simulink model "Temp"  (R2018a)
settings: Solver=FixedStepAuto  StartTime=0.0  StopTime=100  FixedStep=10^-2  RelTol=1e-3
values from neighbouring files (symbols this model uses):
  Af = 80 - ABS_ZERO_TEMP    (= 353.15)    [TempBris.m]    (also in TensileSMA.m = 353)
  As = 70 - ABS_ZERO_TEMP    (= 343.15)    [TempBris.m]    (also in TensileSMA.m = 343)
  austeniteLatentCoef = 12188    [TempBris.m]
  BOLTZ_CONST = 5.6703 * 10^-8    (= 5.6703e-08)    [TempBris.m]
  emissivity = 0.75    [TempBris.m]
  Mf = 40 - ABS_ZERO_TEMP    (= 313.15)    [TempBris.m]    (also in TensileSMA.m = 313)
  Ms = 50 - ABS_ZERO_TEMP    (= 323.15)    [TempBris.m]    (also in TensileSMA.m = 323)
  resistanceAustenite = 4 * pi * wireLength * austeniteResistivity / wireDiameter^2    (= 11.5409547722)    [TempBris.m]
  resistanceMartensite = 4 * pi * wireLength * martensiteResistivity / wireDiameter^2    (= 10.6964946669)    [TempBris.m]
  specificHeat = 465.2    [TempBris.m]
  tempEnd = 80 + 273    (= 353)    [TempBris.m]
  tempStart = 80 + 273    (= 353)    [TempBris.m]
  voltage = 2    [TempBris.m]
  wireMass = wireVolume * density    (= 2.21629544234e-05)    [TempBris.m]
  wireSurfaceArea = wireLength * pi * wireDiameter    (= 5.49778714378e-05)    [TempBris.m]
libraries: simulink x3
settings Model: Creator=Michau  LastModifiedBy=Michau

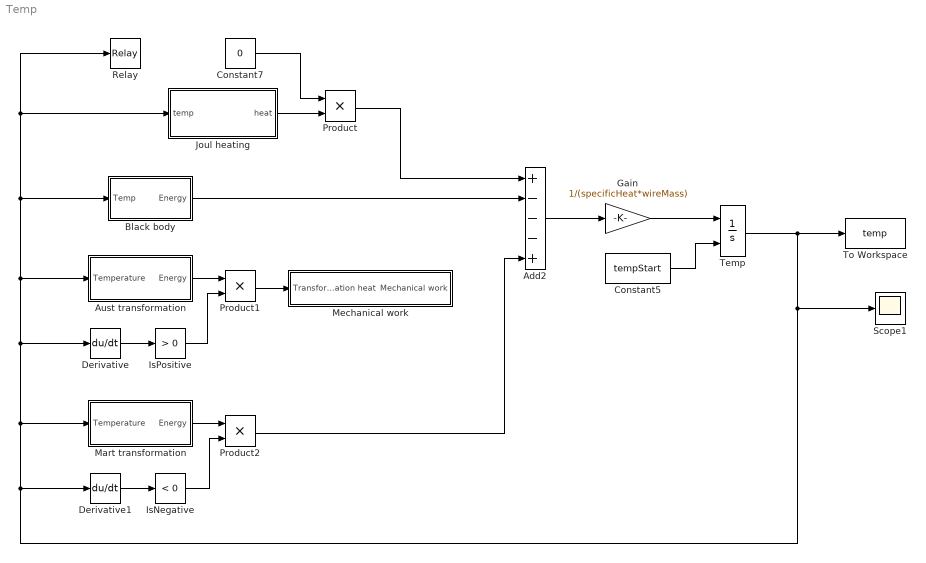
== system Temp ==
  Add2 : Sum  Inputs=+---+
  Aust transformation : Subsystem
  Black body : Subsystem
  Constant5 : Constant  Value=tempStart
  Constant7 : Constant  Value=0
  Derivative : Derivative
  Derivative1 : Derivative
  Gain : Gain  Gain=1/(specificHeat*wireMass)
  IsNegative : simulink/Logic and Bit Operations/Compare To Zero  relop=<  OutDataTypeStr=boolean
  IsPositive : simulink/Logic and Bit Operations/Compare To Zero  relop=>  OutDataTypeStr=boolean
  Joul heating : Subsystem
  Mart transformation : Subsystem
  Mechanical work : Subsystem
  Product : Product
  Product1 : Product
  Product2 : Product
  Relay : Relay  OnSwitchValue=tempEnd+5  OffSwitchValue=tempStart  OnOutputValue=0  OffOutputValue=1
  Scope1 : Scope
  Temp : Integrator  InitialConditionSource=external
  To Workspace : ToWorkspace  VariableName=temp  SaveFormat=Timeseries  SampleTime=-1
  wires:
  Constant5/1 -> Temp/2
  Gain/1 -> Temp/1
  Add2/1 -> Gain/1
  Black body/1(Energy) -> Add2/2
  Joul heating/1(heat) -> Product/2
  Derivative/1 -> IsPositive/1
  IsPositive/1 -> Product1/2
  Aust transformation/1(Energy) -> Product1/1
  Product1/1 -> Mechanical work/1("Transformation heat ")
  Derivative1/1 -> IsNegative/1
  IsNegative/1 -> Product2/2
  Mart transformation/1(Energy) -> Product2/1
  Temp/1 -> Scope1/1, Derivative1/1, Mart transformation/1(Temperature), Aust transformation/1(Temperature), Joul heating/1(temp), Relay/1, Black body/1(Temp), Derivative/1, To Workspace/1
  Product2/1 -> Add2/5
  Constant7/1 -> Product/1
  Product/1 -> Add2/1

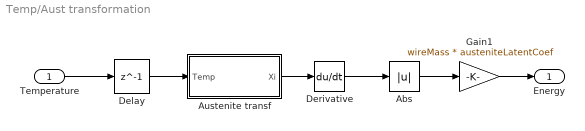
== system Temp/Aust transformation ==
  Temperature : Inport
  Abs : Abs
  Austenite transf : Subsystem
  Delay : Delay  DelayLength=1  InitialCondition=0
  Derivative : Derivative
  Gain1 : Gain  Gain=wireMass * austeniteLatentCoef
  Energy : Outport
  wires:
  Abs/1 -> Gain1/1
  Gain1/1 -> Energy/1
  Austenite transf/1(Xi) -> Derivative/1
  Derivative/1 -> Abs/1
  Delay/1 -> Austenite transf/1(Temp)
  Temperature/1 -> Delay/1

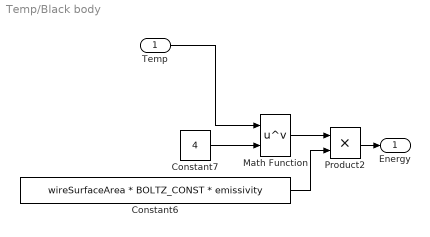
== system Temp/Black body ==
  Temp : Inport
  Constant6 : Constant  Value=wireSurfaceArea * BOLTZ_CONST * emissivity
  Constant7 : Constant  Value=4
  Math Function : Math  Operator=pow  SaturateOnIntegerOverflow=on
  Product2 : Product
  Energy : Outport
  wires:
  Constant7/1 -> Math Function/2
  Temp/1 -> Math Function/1
  Constant6/1 -> Product2/2
  Math Function/1 -> Product2/1
  Product2/1 -> Energy/1

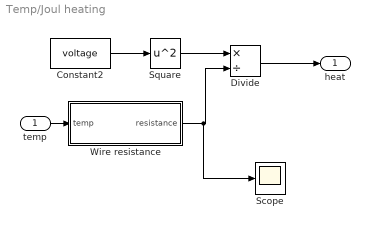
== system Temp/Joul heating ==
  temp : Inport
  Constant2 : Constant  Value=voltage
  Divide : Product  Inputs=*/
  Scope : Scope
  Square : Math  Operator=square  SaturateOnIntegerOverflow=on
  Wire resistance : Subsystem
  heat : Outport
  wires:
  temp/1 -> Wire resistance/1(temp)
  Divide/1 -> heat/1
  Constant2/1 -> Square/1
  Square/1 -> Divide/1
  Wire resistance/1("resistance ") -> Scope/1, Divide/2

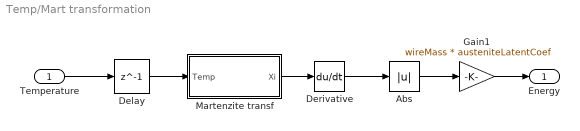
== system Temp/Mart transformation ==
  Temperature : Inport
  Abs : Abs
  Delay : Delay  DelayLength=1  InitialCondition=0
  Derivative : Derivative
  Gain1 : Gain  Gain=wireMass * austeniteLatentCoef
  Martenzite transf : Subsystem
  Energy : Outport
  wires:
  Abs/1 -> Gain1/1
  Gain1/1 -> Energy/1
  Derivative/1 -> Abs/1
  Delay/1 -> Martenzite transf/1(Temp)
  Martenzite transf/1(Xi) -> Derivative/1
  Temperature/1 -> Delay/1

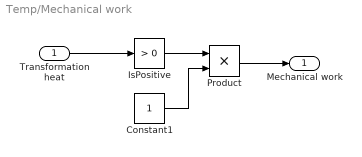
== system Temp/Mechanical work ==
  "Transformation heat " : Inport
  Constant1 : Constant
  IsPositive : simulink/Logic and Bit Operations/Compare To Zero  relop=>  OutDataTypeStr=boolean
  Product : Product
  "Mechanical work " : Outport
  wires:
  Constant1/1 -> Product/2
  Product/1 -> "Mechanical work "/1
  IsPositive/1 -> Product/1
  "Transformation heat "/1 -> IsPositive/1

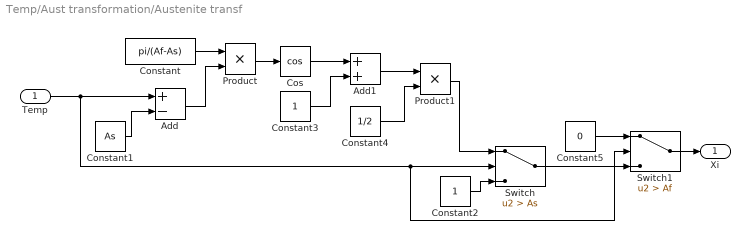
== system Temp/Aust transformation/Austenite transf ==
  Temp : Inport
  Add : Sum  Inputs=+-
  Add1 : Sum
  Constant : Constant  Value=pi/(Af-As)
  Constant1 : Constant  Value=As
  Constant2 : Constant
  Constant3 : Constant
  Constant4 : Constant  Value=1/2
  Constant5 : Constant  Value=0
  Cos : Trigonometry  Operator=cos
  Product : Product
  Product1 : Product
  Switch : Switch  Criteria=u2 > Threshold  Threshold=As
  Switch1 : Switch  Criteria=u2 > Threshold  Threshold=Af
  Xi : Outport
  wires:
  Cos/1 -> Add1/1
  Constant4/1 -> Product1/2
  Constant1/1 -> Add/2
  Product/1 -> Cos/1
  Constant3/1 -> Add1/2
  Add/1 -> Product/2
  Add1/1 -> Product1/1
  Constant/1 -> Product/1
  Product1/1 -> Switch/1
  Constant2/1 -> Switch/3
  Temp/1 -> Switch1/2, Switch/2, Add/1
  Constant5/1 -> Switch1/1
  Switch/1 -> Switch1/3
  Switch1/1 -> Xi/1

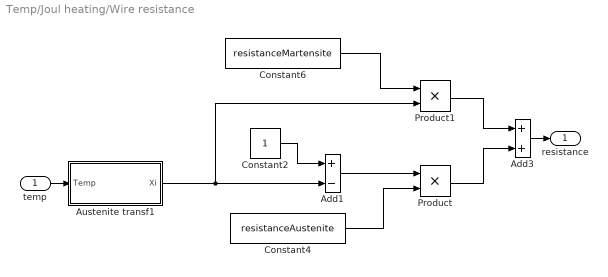
== system Temp/Joul heating/Wire resistance ==
  temp : Inport
  Add1 : Sum  Inputs=+-
  Add3 : Sum
  Austenite transf1 : Subsystem
  Constant2 : Constant
  Constant4 : Constant  Value=resistanceAustenite
  Constant6 : Constant  Value=resistanceMartensite
  Product : Product
  Product1 : Product
  "resistance " : Outport
  wires:
  Austenite transf1/1(Xi) -> Product1/2, Add1/2
  Constant6/1 -> Product1/1
  Constant2/1 -> Add1/1
  Product1/1 -> Add3/1
  temp/1 -> Austenite transf1/1(Temp)
  Constant4/1 -> Product/2
  Add3/1 -> "resistance "/1
  Add1/1 -> Product/1
  Product/1 -> Add3/2

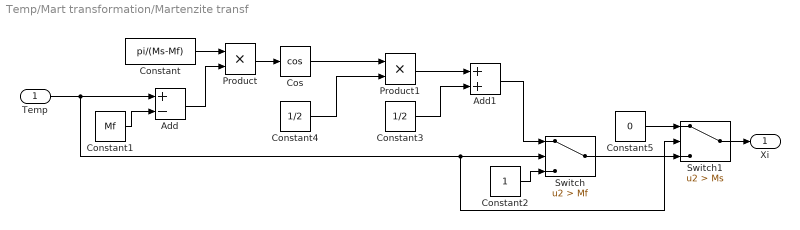
== system Temp/Mart transformation/Martenzite transf ==
  Temp : Inport
  Add : Sum  Inputs=+-
  Add1 : Sum
  Constant : Constant  Value=pi/(Ms-Mf)
  Constant1 : Constant  Value=Mf
  Constant2 : Constant
  Constant3 : Constant  Value=1/2
  Constant4 : Constant  Value=1/2
  Constant5 : Constant  Value=0
  Cos : Trigonometry  Operator=cos
  Product : Product
  Product1 : Product
  Switch : Switch  Criteria=u2 > Threshold  Threshold=Mf
  Switch1 : Switch  Criteria=u2 > Threshold  Threshold=Ms
  Xi : Outport
  wires:
  Constant4/1 -> Product1/2
  Constant1/1 -> Add/2
  Product/1 -> Cos/1
  Add/1 -> Product/2
  Cos/1 -> Product1/1
  Constant/1 -> Product/1
  Constant2/1 -> Switch/3
  Temp/1 -> Switch1/2, Switch/2, Add/1
  Constant5/1 -> Switch1/1
  Switch/1 -> Switch1/3
  Switch1/1 -> Xi/1
  Product1/1 -> Add1/1
  Constant3/1 -> Add1/2
  Add1/1 -> Switch/1

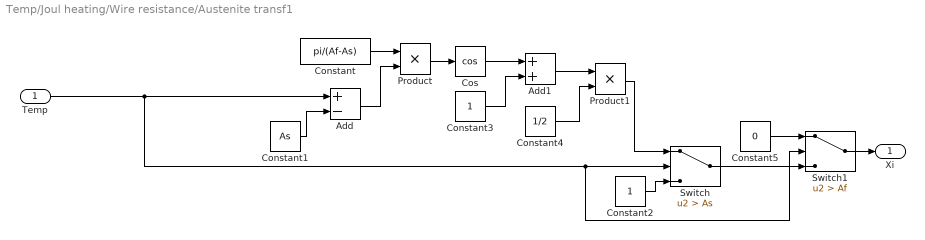
== system Temp/Joul heating/Wire resistance/Austenite transf1 ==
  Temp : Inport
  Add : Sum  Inputs=+-
  Add1 : Sum
  Constant : Constant  Value=pi/(Af-As)
  Constant1 : Constant  Value=As
  Constant2 : Constant
  Constant3 : Constant
  Constant4 : Constant  Value=1/2
  Constant5 : Constant  Value=0
  Cos : Trigonometry  Operator=cos
  Product : Product
  Product1 : Product
  Switch : Switch  Criteria=u2 > Threshold  Threshold=As
  Switch1 : Switch  Criteria=u2 > Threshold  Threshold=Af
  Xi : Outport
  wires:
  Cos/1 -> Add1/1
  Constant4/1 -> Product1/2
  Constant1/1 -> Add/2
  Product/1 -> Cos/1
  Constant3/1 -> Add1/2
  Add/1 -> Product/2
  Add1/1 -> Product1/1
  Constant/1 -> Product/1
  Product1/1 -> Switch/1
  Constant2/1 -> Switch/3
  Temp/1 -> Switch1/2, Switch/2, Add/1
  Constant5/1 -> Switch1/1
  Switch/1 -> Switch1/3
  Switch1/1 -> Xi/1
